simulink model "FSO"  (R2025b)
settings: Solver=VariableStepAuto  StartTime=0.0  StopTime=10  RelTol=1e-3
values from neighbouring files (symbols this model uses):
  A = double(subs(A_sym, sym_vars, num_vals))    [derieve_model.m]    (also in model_data.mat = [0 0 0 0 0 0 1 0 0 0 0 0 ... (36 elements, 6x6)]; pid_controller.m = M1 \ M2)
  B = double(subs(B_sym, sym_vars, num_vals))    [derieve_model.m]    (also in model_data.mat = [0 0.620233683438 0 -3.91197355004 0 0.686278876294]; pid_controller.m = M1 \ M3)
  C = [0 0 1 0 0 0 ... (first row only)    [derieve_model.m]    (also in model_data.mat = [0  0  1  0  0  0; 1  0  0  0  0  0]; pid_controller.m = eye(4))
  fc = 2 * pi * 15    (= 94.2477796077)    [FSO_code.m]    (also in ROO_code.m)
  K = [-1 -5.67883011683 -91.1319066724 -17.4581672697 -52.512729862 -30.6776823134]    [lqr_data.mat]    (also in run_lqr.m = lqr(A, B, Q, R))
  Ke = place(A', C', p_o)'    [FSO_code.m]    (also in ROO_code.m = place(Abb', Aab', p_o)')
  params =     [model_data.mat]
  x0 = [0;                 0;                   deg2rad(15);         0;                   0;                   0]    [FSO_code.m]
  x0_obsv = [0; 0; 0; 0; 0; 0]    [FSO_code.m]
libraries: simulink_extras x2, commchan3 x1
settings Model: Creator=Lenovo  LastModifiedBy=Lenovo

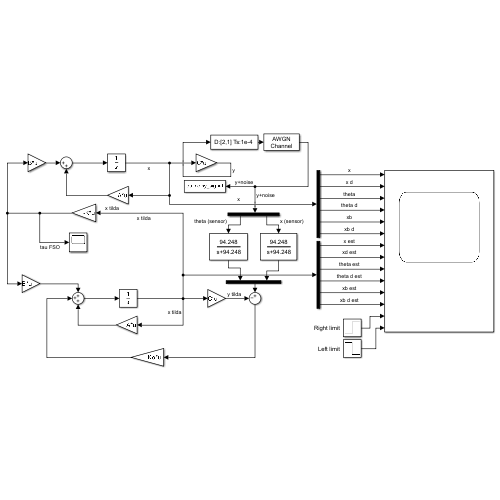
[thumbnail: Simulink's stored preview of the top-level diagram]
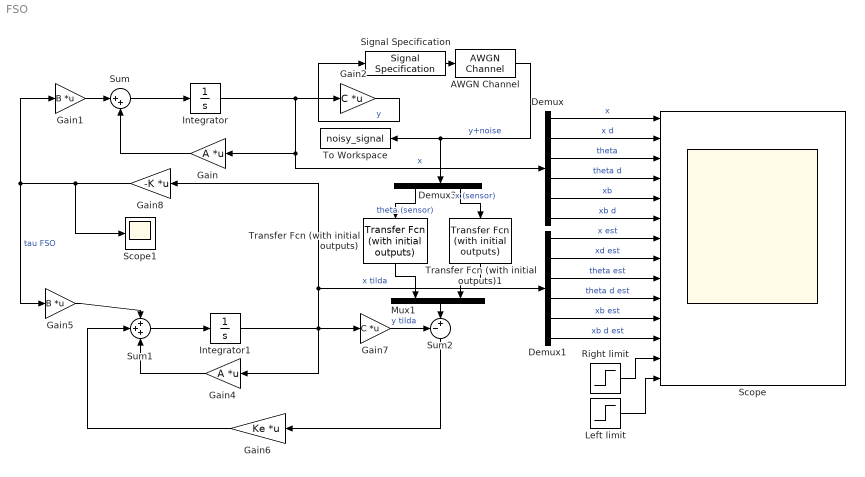
== system FSO ==
  AWGN Channel : commchan3/AWGN Channel  LegacyMode=off  NoiseMethod="Signal to noise ratio  (SNR)"  noiseMode="Signal to noise ratio  (SNR)"  EbNo=10  EsNo=10  SNR=30  BitsPerSymbol=1  SignalPower=1  SpecifySymbolPeriod=off  SamplesPerSymbol=1  SymbolPeriod=1  VarianceSource=Parameter  Variance=1  RandomStream=Global stream  Seed=67  SimulateUsing=Code generation
  Demux : Demux  Outputs=6
  Demux1 : Demux  Outputs=6
  Demux3 : Demux  Outputs=2
  Gain : Gain  Gain=A  Multiplication=Matrix(K*u)
  Gain1 : Gain  Gain=B  Multiplication=Matrix(K*u)
  Gain2 : Gain  Gain=C  Multiplication=Matrix(K*u)
  Gain4 : Gain  Gain=A  Multiplication=Matrix(K*u)
  Gain5 : Gain  Gain=B  Multiplication=Matrix(K*u)
  Gain6 : Gain  Gain=Ke  Multiplication=Matrix(K*u)
  Gain7 : Gain  Gain=C  Multiplication=Matrix(K*u)
  Gain8 : Gain  Gain=-K  Multiplication=Matrix(K*u)
  Integrator : Integrator  InitialCondition=x0
  Integrator1 : Integrator  InitialCondition=x0_obsv
  Left limit : Step  Time=0  After=-params.d/2  SampleTime=0
  Mux1 : Mux  Inputs=2
  Right limit : Step  Time=0  After=params.d/2  SampleTime=0
  Scope : Scope  NumInputPorts=14
      settings: SampleTime=1e-4  ActiveDisplayYMinimum=-0.18004514737433785  ActiveDisplayYMaximum=0.38439971124629296
  Scope1 : Scope
      settings: ActiveDisplayYMinimum=-1  ActiveDisplayYMaximum=1
  Signal Specification : SignalSpecification  Dimensions=[2,1]  SampleTime=1e-4
  Sum : Sum  Inputs=|++
  Sum1 : Sum  Inputs=+++
  Sum2 : Sum  Inputs=-+|
  To Workspace : ToWorkspace  VariableName=noisy_signal  SaveFormat=Structure With Time  SampleTime=1e-4
  Transfer Fcn (with initial outputs) : simulink_extras/Additional Linear/Transfer Fcn (with initial outputs)  N=[fc]  D=[1 fc]  Y0=0  U0=0
  Transfer Fcn (with initial outputs)1 : simulink_extras/Additional Linear/Transfer Fcn (with initial outputs)  N=[fc]  D=[1 fc]  Y0=0  U0=0
  wires:
  Gain/1 -> Sum/2
  Sum/1 -> Integrator/1
  Integrator/1 -> Gain/1, Demux/1, Gain2/1  "x"
  Gain1/1 -> Sum/1
  Gain2/1 -> Signal Specification/1  "y"
  Gain5/1 -> Sum1/1
  Sum1/1 -> Integrator1/1
  Gain4/1 -> Sum1/3
  Gain6/1 -> Sum1/2
  Integrator1/1 -> Gain8/1, Demux1/1, Gain7/1, Gain4/1  "x tilda"
  Gain7/1 -> Sum2/1  "y tilda"
  Sum2/1 -> Gain6/1
  Gain8/1 -> Scope1/1, Gain1/1, Gain5/1  "tau FSO"
  Right limit/1 -> Scope/13
  Left limit/1 -> Scope/14
  Demux/1 -> Scope/1  "x"
  Demux/2 -> Scope/2  "x d"
  Demux1/1 -> Scope/7  "x est"
  Demux1/2 -> Scope/8  "xd est"
  Demux/3 -> Scope/3  "theta"
  Demux/4 -> Scope/4  "theta d"
  Demux/5 -> Scope/5  "xb"
  Demux/6 -> Scope/6  "xb d"
  Demux1/3 -> Scope/9  "theta est"
  Demux1/4 -> Scope/10  "theta d est"
  Demux1/5 -> Scope/11  "xb est"
  Demux1/6 -> Scope/12  "xb d est"
  AWGN Channel/1 -> To Workspace/1, Demux3/1  "y+noise"
  Signal Specification/1 -> AWGN Channel/1
  Demux3/1 -> Transfer Fcn (with initial outputs)/1  "theta (sensor)"
  Transfer Fcn (with initial outputs)/1 -> Mux1/1
  Transfer Fcn (with initial outputs)1/1 -> Mux1/2
  Demux3/2 -> Transfer Fcn (with initial outputs)1/1  "x (sensor)"
  Mux1/1 -> Sum2/2
